simulink model "butterfly_direct_stage_2_test"  (Simulink 7.4)
settings: Solver=VariableStepDiscrete  StartTime=0.0  StopTime=256  RelTol=1e-3
libraries: xbsIndex_r4 x446, casper_library_misc x12
(part 5 of 5)

== system butterfly_direct_stage_2_test/butterfly_direct2/twiddle/pipe_sync ==
  d : Inport
  q : Outport
  wires:
  d/1 -> q/1
